simulink model "TENSGwithGFM_electromechanical"  (R2020a)
settings: Solver=VariableStepAuto  StartTime=0.0  StopTime=10.0  FixedStep=0.01  RelTol=1e-3
values from neighbouring files (symbols this model uses):
  GFMInit = GFMSimple_init(resultsac,GFM_in_gidx)    [init.m]
  GSGInit =     [SixGFMconfig.mat]    (also in eightGFMconfig.mat; fourGFMconfig.mat; init.m = SG_init(resultsac,SG_in_gidx); tenGFMconfig.mat)
  Pload = [0 0 0 0 0 0 0 0 0 0 0 0 ... (39 elements, 39x1)]    [SixGFMconfig.mat]    (also in eightGFMconfig.mat; fourGFMconfig.mat; init.m = -resultsac.bus{[CZno,CPno],3}/1000; tenGFMconfig.mat)
  Qload = -resultsac.bus{[CZno,CPno],4}/1000    [init.m]
  Satura = Ses_g(GFM_in_gidx)    [init.m]
  U = [1.0278659059 0.919047677638 0.824047236404 0.914672565668 0.984993620745 0.992890253418 1.00337242347 1.00687710353 1.06162588537 0.973548635627 0.980333735458 0.971076509646 ... (88 elements, 88x1)]    [SixGFMconfig.mat]    (also in eightGFMconfig.mat; fourGFMconfig.mat; init.m = resultsac.bus{:,8}.*exp(1i*(resultsac.bus{:,9})/180*pi); tenGFMconfig.mat)
  Vload = Vbus([CZno,CPno])    [init.m]
  W0 = wB    (= 314.159265359)    [init.m]
  Y_new = [-5.55111512313e-17 -2.77555756156e-17 0 0 0 0 0 0 0 0 0 0 ... (7744 elements, 88x88)]    [SixGFMconfig.mat]    (also in eightGFMconfig.mat; fourGFMconfig.mat; init.m = Y_new([CSno,CPno,GFMother],[CSno,CPno,GFMother]); kron.m = Y)
libraries: eeTransforms x45, simulink_extras x10
(part 1 of 3)
settings Model: Creator=Qiufan_Yang  LastModifiedBy=Qiufan_Yang
settings SolverCC: ZeroCrossAlgorithm=Adaptive
settings DebuggingCC: IgnoredZcDiagnostic=none

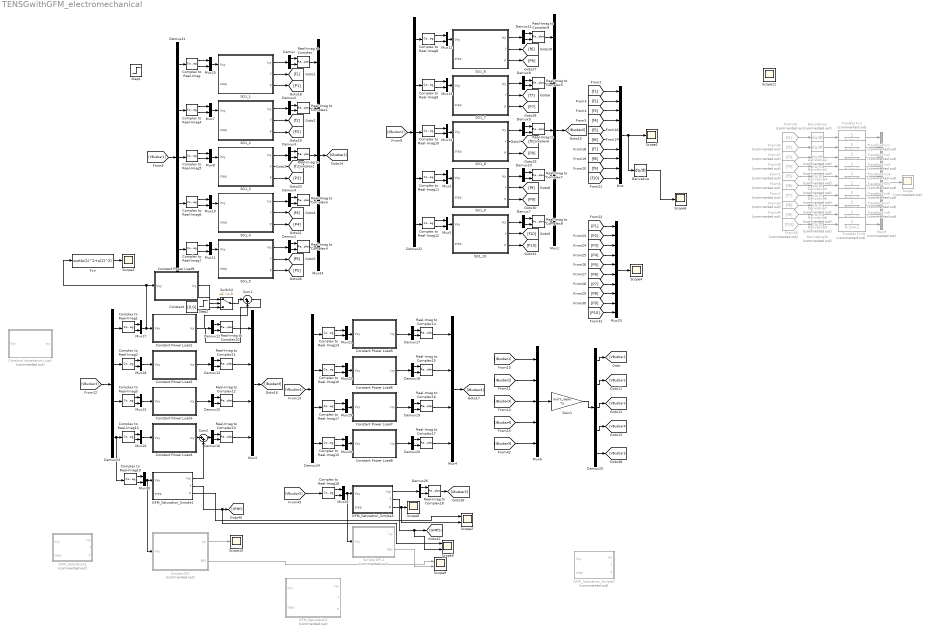
== system TENSGwithGFM_electromechanical ==
  Complex to Real-Imag{,1..19} (20 alike) : ComplexToRealImag
  Constant : Constant  Value=[0,0]
  Constant Impedance Load : Subsystem  Commented=on  mask{Pload=Pload(1), Qload=Qload(1), Vout=Vload(1), Ix0=0, Iy0=0, YLD=0}
      mask init:
      | YLD=(Pload-1j*Qload)/(abs(Vout))^2;
  Constant Power Load1 : Subsystem  mask{Pload=Pload(1), Qload=Qload(1), Vout=Vload(1), Ix0=0, Iy0=0}
      mask init:
      | Ixy=(Pload-1j*Qload)/conj(Vout);
      | Ix0=real(Ixy);
      | Iy0=imag(Ixy);
  Constant Power Load2 : Subsystem  mask{Pload=Pload(2), Qload=Qload(2), Vout=Vload(2), Ix0=0, Iy0=0}
      mask init:
      | Ixy=(Pload-1j*Qload)/conj(Vout);
      | Ix0=real(Ixy);
      | Iy0=imag(Ixy);
  Constant Power Load3 : Subsystem  mask{Pload=Pload(3), Qload=Qload(3), Vout=Vload(3), Ix0=0, Iy0=0}
      mask init:
      | Ixy=(Pload-1j*Qload)/conj(Vout);
      | Ix0=real(Ixy);
      | Iy0=imag(Ixy);
  Constant Power Load4 : Subsystem  mask{Pload=Pload(4), Qload=Qload(4), Vout=Vload(4), Ix0=0, Iy0=0}
      mask init:
      | Ixy=(Pload-1j*Qload)/conj(Vout);
      | Ix0=real(Ixy);
      | Iy0=imag(Ixy);
  Constant Power Load5 : Subsystem  mask{Pload=Pload(5), Qload=Qload(5), Vout=Vload(5), Ix0=0, Iy0=0}
      mask init:
      | Ixy=(Pload-1j*Qload)/conj(Vout);
      | Ix0=real(Ixy);
      | Iy0=imag(Ixy);
  Constant Power Load6 : Subsystem  mask{Pload=Pload(6), Qload=Qload(6), Vout=Vload(6), Ix0=0, Iy0=0}
      mask init:
      | Ixy=(Pload-1j*Qload)/conj(Vout);
      | Ix0=real(Ixy);
      | Iy0=imag(Ixy);
  Constant Power Load7 : Subsystem  mask{Pload=Pload(7), Qload=Qload(7), Vout=Vload(7), Ix0=0, Iy0=0}
      mask init:
      | Ixy=(Pload-1j*Qload)/conj(Vout);
      | Ix0=real(Ixy);
      | Iy0=imag(Ixy);
  Constant Power Load8 : Subsystem  mask{Pload=Pload(8), Qload=Qload(8), Vout=Vload(8), Ix0=0, Iy0=0}
      mask init:
      | Ixy=(Pload-1j*Qload)/conj(Vout);
      | Ix0=real(Ixy);
      | Iy0=imag(Ixy);
  Constant Power Load9 : Subsystem  mask{Pload=-0.2, Qload=0, Vout=Vload(1), Ix0=0, Iy0=0}
      mask init:
      | Ixy=(Pload-1j*Qload)/conj(Vout);
      | Ix0=real(Ixy);
      | Iy0=imag(Ixy);
  Demux{,1..4,7..13,15..20,26} (19 alike) : Demux  Outputs=2
  Demux21 : Demux  Outputs=5
  Demux22 : Demux  Outputs=5
  Demux23 : Demux
  Demux24 : Demux
  Demux25 : Demux  Outputs=[5 5 4 4 1]
  Derivative : Derivative  CoefficientInTFapproximation=1
  Derivative{1..10} (10 alike) : Derivative  Commented=on
  Fcn : Fcn  Expr=sqrt(u(1)^2+u(2)^2)
  From1 : From  Commented=on  GotoTag=f5
  From32 : From  Commented=on  GotoTag=f8
  From33 : From  Commented=on  GotoTag=f1
  From34 : From  Commented=on  GotoTag=f9
  From35 : From  Commented=on  GotoTag=f10
  From36 : From  Commented=on  GotoTag=f2
  From37 : From  Commented=on  GotoTag=f3
  From38 : From  Commented=on  GotoTag=f4
  From6 : From  Commented=on  GotoTag=f6
  From7 : From  Commented=on  GotoTag=f7
  GFM_Saturation1 : Subsystem  Commented=on  mask{Pout=1, Qout=0, Vout=1, RG=GFMInit.RG(1), LG=GFMInit.LG(1), CF=GFMInit.CF(1), LF=GFMInit.LF(1), RF=GFMInit.RF(1), JGFM=GFMInit.J(1), DGFM=GFMInit.D(1), KPV=GFMInit.KPV(1), KIV=GFMInit.KIV(1), KIF=GFMInit.KIF(1), KPC=GFMInit.KPC(1), KIC=GFMInit.KIC(1), KVF=GFMInit.KVF(1), TVF=GFMInit.TVF(1), Pref=GFMInit.Pref(1), Qref=GFMInit.Qref(1), Vd0=GFMInit.Vd0(1), theta0=GFMInit.theta0(1), Ix0=GFMInit.Ix0(1), Iy0=GFMInit.Iy0(1), Vx0=GFMInit.Vx0(1), Vy0=GFMInit.Vy0(1), IOx0=GFMInit.IOx0(1), IOy0=GFMInit.IOy0(1), Idref0=GFMInit.Idref0(1), Iqref0=GFMInit.Iqref0(1), Ed0=GFMInit.Ed0(1), Eq0=GFMInit.Eq0(1), Plimit=Satura(1)*1000, Qreflimit=0, KPLlimit=0.16*10, KILlimit=13.26, Ix0_copy=0.5, Iy0_copy=10}
      mask prompts: Qreflimit "Qlimit"; Ix0_copy "KPPlimit"; Iy0_copy "KIPlimit"
      mask init:
      | %IOxy0 = (Pout - 1i*Qout)/conj(Vout);
      | %Vxy0  = Vout + IOxy0*(RG+1i*LG);
      | %Ixy0  = IOxy0 + Vxy0*(1i*CF);
      | %Exy0  = Vxy0 + Ixy0*(RF+1i*LF);
      | 
      | %IOx0 = real(IOxy0);
      | % IOy0 = imag(IOxy0);
      | % Vx0 = real(Vxy0);
      | % Vy0 = imag(Vxy0);
      | % Ix0 = real(Ixy0);
      | % Iy0 = imag(Ixy0);
      | % Pref = real(Vxy0*conj(IOxy0));
      | % Qref = imag(Vxy0*conj(IOxy0));
      | % Vd0  = abs(Vxy0);
      | % theta0 = angle(Vxy0);
      | % 
      | % Edq0 = abs(Exy0)*exp(1i*(angle(Exy0)-theta0));
      | % Idq0 = abs(Ixy0)*exp(1i*(angle(Ixy0)-theta0));
      | % IOdq0 = abs(IOxy0)*exp(1i*(angle(IOxy0)-theta0));
      | % 
      | % temp = Edq0 - KVF*Vd0 - Idq0*(1i*LF);
      | % Ed0 = real(temp);
      | % Eq0 = imag(temp);
      | % 
      | % temp = Idq0 - KIF*IOdq0 - Vd0*(1i*CF);
      | % Idref0 = real(temp);
      | % Iqref0 = imag(temp);
      mask DialogControl Container8 Prompt: Parameters
      mask DialogControl Container9 Prompt: Power Flow
      mask DialogControl Container10 Prompt: LCL Parameters
      mask DialogControl Container20 Prompt: Control Parameters
      mask DialogControl Container21 Prompt: Initial Parameters
      mask DialogControl Container22 Prompt: Saturation Parameters
  GFM_Saturation2 : Subsystem  Commented=on  mask{Pout=1, Qout=0, Vout=1, RG=GFMInit.RG(2), LG=GFMInit.LG(2), CF=GFMInit.CF(2), LF=GFMInit.LF(2), RF=GFMInit.RF(2), JGFM=GFMInit.J(2), DGFM=GFMInit.D(2), KPV=GFMInit.KPV(2), KIV=GFMInit.KIV(2), KIF=GFMInit.KIF(2), KPC=GFMInit.KPC(2), KIC=GFMInit.KIC(2), KVF=GFMInit.KVF(2), TVF=GFMInit.TVF(2), Pref=GFMInit.Pref(2), Qref=GFMInit.Qref(2), Vd0=GFMInit.Vd0(2), theta0=GFMInit.theta0(2), Ix0=GFMInit.Ix0(2), Iy0=GFMInit.Iy0(2), Vx0=GFMInit.Vx0(2), Vy0=GFMInit.Vy0(2), IOx0=GFMInit.IOx0(2), IOy0=GFMInit.IOy0(2), Idref0=GFMInit.Idref0(2), Iqref0=GFMInit.Iqref0(2), Ed0=GFMInit.Ed0(2), Eq0=GFMInit.Eq0(2), Plimit=Satura(2)*1000, Qreflimit=0, KPLlimit=0.16*10, KILlimit=13.26, Ix0_copy=0.5, Iy0_copy=10}
      mask prompts: Qreflimit "Qlimit"; Ix0_copy "KPPlimit"; Iy0_copy "KIPlimit"
      mask init: same as TENSGwithGFM_electromechanical/GFM_Saturation1
      mask DialogControl Container8 Prompt: Parameters
      mask DialogControl Container9 Prompt: Power Flow
      mask DialogControl Container10 Prompt: LCL Parameters
      mask DialogControl Container20 Prompt: Control Parameters
      mask DialogControl Container21 Prompt: Initial Parameters
      mask DialogControl Container22 Prompt: Saturation Parameters
  GFM_Saturation_Simple1 : Subsystem  mask{Pout=0, Qout=0, Vout=Vload(4), Pref=0, theta0=GFMInit.theta0(1), EQ=GFMInit.EQ(1), LG=GFMInit.LG(1), JGFM=GFMInit.J(1)*0+0.5742, DGFM=GFMInit.D(1), Plimit=Satura(1)*0+0.05742, Qreflimit=0, KPLlimit=0.16*10, KILlimit=13.26, Ix0_copy=0.5, Iy0_copy=10}
      mask prompts: Qreflimit "Qlimit"; Ix0_copy "KPPlimit"; Iy0_copy "KIPlimit"
      mask init: same as TENSGwithGFM_electromechanical/GFM_Saturation1
      mask DialogControl Container8 Prompt: Parameters
      mask DialogControl Container9 Prompt: Power Flow
      mask DialogControl Container10 Prompt: LCL Parameters
      mask DialogControl Container20 Prompt: Control Parameters
      mask DialogControl Container22 Prompt: Saturation Parameters
  GFM_Saturation_Simple2 : Subsystem  Commented=on  mask{Pout=1, Qout=0, Vout=1, RG=GFMInit.RG(2), LG=GFMInit.LG(2), CF=GFMInit.CF(2), LF=GFMInit.LF(2), RF=GFMInit.RF(2), JGFM=GFMInit.J(2), DGFM=GFMInit.D(2), KPV=GFMInit.KPV(2), KIV=GFMInit.KIV(2), KIF=GFMInit.KIF(2), KPC=GFMInit.KPC(2), KIC=GFMInit.KIC(2), KVF=GFMInit.KVF(2), TVF=GFMInit.TVF(2), Pref=GFMInit.Pref(2), Qref=GFMInit.Qref(2), Vd0=GFMInit.Vd0(2), theta0=GFMInit.theta0(2), Ix0=GFMInit.Ix0(2), Iy0=GFMInit.Iy0(2), Vx0=GFMInit.Vx0(2), Vy0=GFMInit.Vy0(2), IOx0=GFMInit.IOx0(2), IOy0=GFMInit.IOy0(2), Idref0=GFMInit.Idref0(2), Iqref0=GFMInit.Iqref0(2), Ed0=GFMInit.Ed0(2), Eq0=GFMInit.Eq0(2), Plimit=Satura(2)*1000, Qreflimit=0, KPLlimit=0.16*10, KILlimit=13.26, Ix0_copy=0.5, Iy0_copy=10}
      mask prompts: Qreflimit "Qlimit"; Ix0_copy "KPPlimit"; Iy0_copy "KIPlimit"
      mask init: same as TENSGwithGFM_electromechanical/GFM_Saturation1
      mask DialogControl Container8 Prompt: Parameters
      mask DialogControl Container9 Prompt: Power Flow
      mask DialogControl Container10 Prompt: LCL Parameters
      mask DialogControl Container20 Prompt: Control Parameters
      mask DialogControl Container21 Prompt: Initial Parameters
      mask DialogControl Container22 Prompt: Saturation Parameters
  GFM_Saturation_Simple3 : Subsystem  mask{Pout=0, Qout=0, Vout=U(22), Pref=0, theta0=GFMInit.theta0(2), EQ=GFMInit.EQ(2), LG=GFMInit.LG(2), JGFM=GFMInit.J(2)*0+0.6571, DGFM=GFMInit.D(2), Plimit=Satura(2)*0+0.059, Qreflimit=0, KPLlimit=0.16*10, KILlimit=13.26, Ix0_copy=0.5, Iy0_copy=10}
      mask prompts: Qreflimit "Qlimit"; Ix0_copy "KPPlimit"; Iy0_copy "KIPlimit"
      mask init: same as TENSGwithGFM_electromechanical/GFM_Saturation1
      mask DialogControl Container8 Prompt: Parameters
      mask DialogControl Container9 Prompt: Power Flow
      mask DialogControl Container10 Prompt: LCL Parameters
      mask DialogControl Container20 Prompt: Control Parameters
      mask DialogControl Container22 Prompt: Saturation Parameters
  Gain1 : Gain  Gain=inv(Y_new)  Multiplication=Matrix(K*u)
  Mux : Mux  Inputs=10
  Mux1 : Mux  Inputs=5
  Mux{2,5,7..8,10..22,25,29..30} (20 alike) : Mux  Inputs=2
  Mux23 : Mux  Inputs=10
  Mux24 : Mux  Inputs=5
  Mux3 : Mux
  Mux4 : Mux
  Mux6 : Mux  Inputs=5
  Mux9 : Mux  Commented=on  Inputs=10
  Real-Imag to Complex{,1..18} (19 alike) : RealImagToComplex
  SG1_1 : Subsystem  mask{Pout=1, Qout=0, Vout=1, RG=0, LG=0, Xd=GSGInit.Xd(1), Xd1=GSGInit.Xd1(1), Xq=GSGInit.Xq(1), Td1=GSGInit.Td1(1), KAVR=GSGInit.KAVR(1), TAVR=GSGInit.TAVR(1), JSG=GSGInit.J(1), DSG=GSGInit.D(1), Ksg=GSGInit.Ksg(1), K1=GSGInit.K1(1), K3=GSGInit.K3(1), K5=GSGInit.K5(1), K7=GSGInit.K7(1), T1=GSGInit.T1(1), T2=GSGInit.T2(1), T3=GSGInit.T3(1), T4=GSGInit.T4(1), T5=GSGInit.T5(1), T6=GSGInit.T6(1), T7=GSGInit.T7(1), Pref=GSGInit.Pref(1), Efd0=GSGInit.Efd0(1), theta0=GSGInit.theta0(1), Eq10=GSGInit.Eq10(1), Vref0=GSGInit.Vref0(1)}
      mask init:
      | % IOxy0 = (Pout - 1i*Qout)/conj(Vout);
      | % % Vxy0  = Vout + IOxy0*(RG+1i*LG);
      | % EQ = Vout + 1i*Xq*IOxy0;
      | % 
      | % Vd = abs(Vout)*sin(angle(EQ)-angle(Vout));
      | % Vq = abs(Vout)*cos(angle(EQ)-angle(Vout));
      | % Iq = Vd/Xq;
      | % Id = abs(IOxy0)*sin(angle(EQ) - angle(IOxy0));
      | % 
      | % theta0 = angle(EQ) - pi/2; 
      | % 
      | % 
      | % Pref = real(Vout*conj(IOxy0));
      | % Qref = imag(Vout*conj(IOxy0));
      | % IOx0 = real(IOxy0);
      | % IOy0 = imag(IOxy0);
      | % 
      | % Eq10 = Vq + Id*Xd1;
      | % 
      | % Efd0 = Eq10 + Id*(Xd-Xd1);
      | % Vref0  = Efd0/KAVR+abs(Vout);
      | %Efd0 = Efd/KAVR;
      mask DialogControl Container8 Prompt: Parameters
      mask DialogControl Container9 Prompt: Power Flow
      mask DialogControl Container10 Prompt: L Parameters
      mask DialogControl Container12 Prompt: Transient Parameter
      mask DialogControl Container20 Prompt: Control Parameters
      mask DialogControl Container14 Prompt: AVR
      mask DialogControl Container16 Prompt: Swing
      mask DialogControl Container15 Prompt: Governor
      mask DialogControl Container21 Prompt: Initial Parameters
  SG1_10 : Subsystem  mask{Pout=1, Qout=0, Vout=1, RG=0, LG=0, Xd=GSGInit.Xd(10), Xd1=GSGInit.Xd1(10), Xq=GSGInit.Xq(10), Td1=GSGInit.Td1(10), KAVR=GSGInit.KAVR(10), TAVR=GSGInit.TAVR(10), JSG=GSGInit.J(10), DSG=GSGInit.D(10), Ksg=GSGInit.Ksg(10), K1=GSGInit.K1(10), K3=GSGInit.K3(10), K5=GSGInit.K5(10), K7=GSGInit.K7(10), T1=GSGInit.T1(10), T2=GSGInit.T2(10), T3=GSGInit.T3(10), T4=GSGInit.T4(10), T5=GSGInit.T5(10), T6=GSGInit.T6(10), T7=GSGInit.T7(10), Pref=GSGInit.Pref(10), Efd0=GSGInit.Efd0(10), theta0=GSGInit.theta0(10), Eq10=GSGInit.Eq10(10), Vref0=GSGInit.Vref0(10)}
      mask init: same as TENSGwithGFM_electromechanical/SG1_1
      mask DialogControl Container8 Prompt: Parameters
      mask DialogControl Container9 Prompt: Power Flow
      mask DialogControl Container10 Prompt: L Parameters
      mask DialogControl Container12 Prompt: Transient Parameter
      mask DialogControl Container20 Prompt: Control Parameters
      mask DialogControl Container14 Prompt: AVR
      mask DialogControl Container16 Prompt: Swing
      mask DialogControl Container15 Prompt: Governor
      mask DialogControl Container21 Prompt: Initial Parameters
  SG1_2 : Subsystem  mask{Pout=1, Qout=0, Vout=1, RG=0, LG=0, Xd=GSGInit.Xd(2), Xd1=GSGInit.Xd1(2), Xq=GSGInit.Xq(2), Td1=GSGInit.Td1(2), KAVR=GSGInit.KAVR(2), TAVR=GSGInit.TAVR(2), JSG=GSGInit.J(2), DSG=GSGInit.D(2), Ksg=GSGInit.Ksg(2), K1=GSGInit.K1(2), K3=GSGInit.K3(2), K5=GSGInit.K5(2), K7=GSGInit.K7(2), T1=GSGInit.T1(2), T2=GSGInit.T2(2), T3=GSGInit.T3(2), T4=GSGInit.T4(2), T5=GSGInit.T5(2), T6=GSGInit.T6(2), T7=GSGInit.T7(2), Pref=GSGInit.Pref(2), Efd0=GSGInit.Efd0(2), theta0=GSGInit.theta0(2), Eq10=GSGInit.Eq10(2), Vref0=GSGInit.Vref0(2)}
      mask init: same as TENSGwithGFM_electromechanical/SG1_1
      mask DialogControl Container8 Prompt: Parameters
      mask DialogControl Container9 Prompt: Power Flow
      mask DialogControl Container10 Prompt: L Parameters
      mask DialogControl Container12 Prompt: Transient Parameter
      mask DialogControl Container20 Prompt: Control Parameters
      mask DialogControl Container14 Prompt: AVR
      mask DialogControl Container16 Prompt: Swing
      mask DialogControl Container15 Prompt: Governor
      mask DialogControl Container21 Prompt: Initial Parameters
  SG1_3 : Subsystem  mask{Pout=1, Qout=0, Vout=1, RG=0, LG=0, Xd=GSGInit.Xd(3), Xd1=GSGInit.Xd1(3), Xq=GSGInit.Xq(3), Td1=GSGInit.Td1(3), KAVR=GSGInit.KAVR(3), TAVR=GSGInit.TAVR(3), JSG=GSGInit.J(3), DSG=GSGInit.D(3), Ksg=GSGInit.Ksg(3), K1=GSGInit.K1(3), K3=GSGInit.K3(3), K5=GSGInit.K5(3), K7=GSGInit.K7(3), T1=GSGInit.T1(3), T2=GSGInit.T2(3), T3=GSGInit.T3(3), T4=GSGInit.T4(3), T5=GSGInit.T5(3), T6=GSGInit.T6(3), T7=GSGInit.T7(3), Pref=GSGInit.Pref(3), Efd0=GSGInit.Efd0(3), theta0=GSGInit.theta0(3), Eq10=GSGInit.Eq10(3), Vref0=GSGInit.Vref0(3)}
      mask init: same as TENSGwithGFM_electromechanical/SG1_1
      mask DialogControl Container8 Prompt: Parameters
      mask DialogControl Container9 Prompt: Power Flow
      mask DialogControl Container10 Prompt: L Parameters
      mask DialogControl Container12 Prompt: Transient Parameter
      mask DialogControl Container20 Prompt: Control Parameters
      mask DialogControl Container14 Prompt: AVR
      mask DialogControl Container16 Prompt: Swing
      mask DialogControl Container15 Prompt: Governor
      mask DialogControl Container21 Prompt: Initial Parameters
  SG1_4 : Subsystem  mask{Pout=1, Qout=0, Vout=1, RG=0, LG=0, Xd=GSGInit.Xd(4), Xd1=GSGInit.Xd1(4), Xq=GSGInit.Xq(4), Td1=GSGInit.Td1(4), KAVR=GSGInit.KAVR(4), TAVR=GSGInit.TAVR(4), JSG=GSGInit.J(4), DSG=GSGInit.D(4), Ksg=GSGInit.Ksg(4), K1=GSGInit.K1(4), K3=GSGInit.K3(4), K5=GSGInit.K5(4), K7=GSGInit.K7(4), T1=GSGInit.T1(4), T2=GSGInit.T2(4), T3=GSGInit.T3(4), T4=GSGInit.T4(4), T5=GSGInit.T5(4), T6=GSGInit.T6(4), T7=GSGInit.T7(4), Pref=GSGInit.Pref(4), Efd0=GSGInit.Efd0(4), theta0=GSGInit.theta0(4), Eq10=GSGInit.Eq10(4), Vref0=GSGInit.Vref0(4)}
      mask init: same as TENSGwithGFM_electromechanical/SG1_1
      mask DialogControl Container8 Prompt: Parameters
      mask DialogControl Container9 Prompt: Power Flow
      mask DialogControl Container10 Prompt: L Parameters
      mask DialogControl Container12 Prompt: Transient Parameter
      mask DialogControl Container20 Prompt: Control Parameters
      mask DialogControl Container14 Prompt: AVR
      mask DialogControl Container16 Prompt: Swing
      mask DialogControl Container15 Prompt: Governor
      mask DialogControl Container21 Prompt: Initial Parameters
  SG1_5 : Subsystem  mask{Pout=1, Qout=0, Vout=1, RG=0, LG=0, Xd=GSGInit.Xd(5), Xd1=GSGInit.Xd1(5), Xq=GSGInit.Xq(5), Td1=GSGInit.Td1(5), KAVR=GSGInit.KAVR(5), TAVR=GSGInit.TAVR(5), JSG=GSGInit.J(5), DSG=GSGInit.D(5), Ksg=GSGInit.Ksg(5), K1=GSGInit.K1(5), K3=GSGInit.K3(5), K5=GSGInit.K5(5), K7=GSGInit.K7(5), T1=GSGInit.T1(5), T2=GSGInit.T2(5), T3=GSGInit.T3(5), T4=GSGInit.T4(5), T5=GSGInit.T5(5), T6=GSGInit.T6(5), T7=GSGInit.T7(5), Pref=GSGInit.Pref(5), Efd0=GSGInit.Efd0(5), theta0=GSGInit.theta0(5), Eq10=GSGInit.Eq10(5), Vref0=GSGInit.Vref0(5)}
      mask init: same as TENSGwithGFM_electromechanical/SG1_1
      mask DialogControl Container8 Prompt: Parameters
      mask DialogControl Container9 Prompt: Power Flow
      mask DialogControl Container10 Prompt: L Parameters
      mask DialogControl Container12 Prompt: Transient Parameter
      mask DialogControl Container20 Prompt: Control Parameters
      mask DialogControl Container14 Prompt: AVR
      mask DialogControl Container16 Prompt: Swing
      mask DialogControl Container15 Prompt: Governor
      mask DialogControl Container21 Prompt: Initial Parameters
  SG1_6 : Subsystem  mask{Pout=1, Qout=0, Vout=1, RG=0, LG=0, Xd=GSGInit.Xd(6), Xd1=GSGInit.Xd1(6), Xq=GSGInit.Xq(6), Td1=GSGInit.Td1(6), KAVR=GSGInit.KAVR(6), TAVR=GSGInit.TAVR(6), JSG=GSGInit.J(6), DSG=GSGInit.D(6), Ksg=GSGInit.Ksg(6), K1=GSGInit.K1(6), K3=GSGInit.K3(6), K5=GSGInit.K5(6), K7=GSGInit.K7(6), T1=GSGInit.T1(6), T2=GSGInit.T2(6), T3=GSGInit.T3(6), T4=GSGInit.T4(6), T5=GSGInit.T5(6), T6=GSGInit.T6(6), T7=GSGInit.T7(6), Pref=GSGInit.Pref(6), Efd0=GSGInit.Efd0(6), theta0=GSGInit.theta0(6), Eq10=GSGInit.Eq10(6), Vref0=GSGInit.Vref0(6)}
      mask init: same as TENSGwithGFM_electromechanical/SG1_1
      mask DialogControl Container8 Prompt: Parameters
      mask DialogControl Container9 Prompt: Power Flow
      mask DialogControl Container10 Prompt: L Parameters
      mask DialogControl Container12 Prompt: Transient Parameter
      mask DialogControl Container20 Prompt: Control Parameters
      mask DialogControl Container14 Prompt: AVR
      mask DialogControl Container16 Prompt: Swing
      mask DialogControl Container15 Prompt: Governor
      mask DialogControl Container21 Prompt: Initial Parameters
  SG1_7 : Subsystem  mask{Pout=1, Qout=0, Vout=1, RG=0, LG=0, Xd=GSGInit.Xd(7), Xd1=GSGInit.Xd1(7), Xq=GSGInit.Xq(7), Td1=GSGInit.Td1(7), KAVR=GSGInit.KAVR(7), TAVR=GSGInit.TAVR(7), JSG=GSGInit.J(7), DSG=GSGInit.D(7), Ksg=GSGInit.Ksg(7), K1=GSGInit.K1(7), K3=GSGInit.K3(7), K5=GSGInit.K5(7), K7=GSGInit.K7(7), T1=GSGInit.T1(7), T2=GSGInit.T2(7), T3=GSGInit.T3(7), T4=GSGInit.T4(7), T5=GSGInit.T5(7), T6=GSGInit.T6(7), T7=GSGInit.T7(7), Pref=GSGInit.Pref(7), Efd0=GSGInit.Efd0(7), theta0=GSGInit.theta0(7), Eq10=GSGInit.Eq10(7), Vref0=GSGInit.Vref0(7)}
      mask init: same as TENSGwithGFM_electromechanical/SG1_1
      mask DialogControl Container8 Prompt: Parameters
      mask DialogControl Container9 Prompt: Power Flow
      mask DialogControl Container10 Prompt: L Parameters
      mask DialogControl Container12 Prompt: Transient Parameter
      mask DialogControl Container20 Prompt: Control Parameters
      mask DialogControl Container14 Prompt: AVR
      mask DialogControl Container16 Prompt: Swing
      mask DialogControl Container15 Prompt: Governor
      mask DialogControl Container21 Prompt: Initial Parameters
  SG1_8 : Subsystem  mask{Pout=1, Qout=0, Vout=1, RG=0, LG=0, Xd=GSGInit.Xd(8), Xd1=GSGInit.Xd1(8), Xq=GSGInit.Xq(8), Td1=GSGInit.Td1(8), KAVR=GSGInit.KAVR(8), TAVR=GSGInit.TAVR(8), JSG=GSGInit.J(8), DSG=GSGInit.D(8), Ksg=GSGInit.Ksg(8), K1=GSGInit.K1(8), K3=GSGInit.K3(8), K5=GSGInit.K5(8), K7=GSGInit.K7(8), T1=GSGInit.T1(8), T2=GSGInit.T2(8), T3=GSGInit.T3(8), T4=GSGInit.T4(8), T5=GSGInit.T5(8), T6=GSGInit.T6(8), T7=GSGInit.T7(8), Pref=GSGInit.Pref(8), Efd0=GSGInit.Efd0(8), theta0=GSGInit.theta0(8), Eq10=GSGInit.Eq10(8), Vref0=GSGInit.Vref0(8)}
      mask init: same as TENSGwithGFM_electromechanical/SG1_1
      mask DialogControl Container8 Prompt: Parameters
      mask DialogControl Container9 Prompt: Power Flow
      mask DialogControl Container10 Prompt: L Parameters
      mask DialogControl Container12 Prompt: Transient Parameter
      mask DialogControl Container20 Prompt: Control Parameters
      mask DialogControl Container14 Prompt: AVR
      mask DialogControl Container16 Prompt: Swing
      mask DialogControl Container15 Prompt: Governor
      mask DialogControl Container21 Prompt: Initial Parameters
  SG1_9 : Subsystem  mask{Pout=1, Qout=0, Vout=1, RG=0, LG=0, Xd=GSGInit.Xd(9), Xd1=GSGInit.Xd1(9), Xq=GSGInit.Xq(9), Td1=GSGInit.Td1(9), KAVR=GSGInit.KAVR(9), TAVR=GSGInit.TAVR(9), JSG=GSGInit.J(9), DSG=GSGInit.D(9), Ksg=GSGInit.Ksg(9), K1=GSGInit.K1(9), K3=GSGInit.K3(9), K5=GSGInit.K5(9), K7=GSGInit.K7(9), T1=GSGInit.T1(9), T2=GSGInit.T2(9), T3=GSGInit.T3(9), T4=GSGInit.T4(9), T5=GSGInit.T5(9), T6=GSGInit.T6(9), T7=GSGInit.T7(9), Pref=GSGInit.Pref(9), Efd0=GSGInit.Efd0(9), theta0=GSGInit.theta0(9), Eq10=GSGInit.Eq10(9), Vref0=GSGInit.Vref0(9)}
      mask init: same as TENSGwithGFM_electromechanical/SG1_1
      mask DialogControl Container8 Prompt: Parameters
      mask DialogControl Container9 Prompt: Power Flow
      mask DialogControl Container10 Prompt: L Parameters
      mask DialogControl Container12 Prompt: Transient Parameter
      mask DialogControl Container20 Prompt: Control Parameters
      mask DialogControl Container14 Prompt: AVR
      mask DialogControl Container16 Prompt: Swing
      mask DialogControl Container15 Prompt: Governor
      mask DialogControl Container21 Prompt: Initial Parameters
  Scope : Scope  Commented=on
  Scope{1,3..4,6,8,10} (6 alike) : Scope
  Scope{2,5,9,11} (4 alike) : Scope  NumInputPorts=2
  Simple GFL : Subsystem  Commented=on  mask{JGFL=GFMInit.J(1)*0, DGFL=GFMInit.D(1)*0, KP=0.16, KI=3.71, TF=0.01, TD=0.01, TO=0.1, Pref=0, Qref=0, Id0=0, Iq0=0, theta=angle(Vload(4))}
  Simple GFL1 : Subsystem  Commented=on  mask{JGFL=GFMInit.J(2)*0, DGFL=GFMInit.D(2)*0, KP=0.16, KI=3.71, TF=0.01, TD=0.01, TO=0.1, Pref=0, Qref=0, Id0=0, Iq0=0, theta=angle(U(22))}
  Step1 : Step  After=-0.1  SampleTime=0
  Step2 : Step  SampleTime=0
  Sum1 : Sum  Inputs=|++
  Sum2 : Sum  Inputs=|++
  Switch2 : Switch  Criteria=u2 ~= 0  Threshold=0.5  SaturateOnIntegerOverflow=on
  Transfer Fcn{,1..9} (10 alike) : TransferFcn  Commented=on  Denominator=[0.1 1]
  wires:
  SG1_1/1(Ixy) -> Demux/1
  SG1_4/1(Ixy) -> Demux4/1
  Real-Imag to Complex/1 -> Mux24/1
  Real-Imag to Complex3/1 -> Mux24/4
  SG1_1/2(f) -> [f1]
  Demux/2 -> Real-Imag to Complex/2
  SG1_3/1(Ixy) -> Demux3/1
  SG1_1/3(P) -> [P1]
  Demux4/1 -> Real-Imag to Complex3/1
  Demux2/2 -> Real-Imag to Complex1/2
  Real-Imag to Complex1/1 -> Mux24/2
  Demux/1 -> Real-Imag to Complex/1
  Real-Imag to Complex2/1 -> Mux24/3
  Demux2/1 -> Real-Imag to Complex1/1
  Demux3/2 -> Real-Imag to Complex2/2
  SG1_2/1(Ixy) -> Demux2/1
  Demux4/2 -> Real-Imag to Complex3/2
  Demux3/1 -> Real-Imag to Complex2/1
  SG1_2/2(f) -> [f2]
  SG1_3/2(f) -> [f3]
  SG1_4/2(f) -> [f4]
  [f1] -> Mux/1
  [f2] -> Mux/2
  [f3] -> Mux/3
  [f4] -> Mux/4
  Mux/1 -> Derivative/1, Scope1/1
  SG1_5/2(f) -> [f5]
  SG1_5/1(Ixy) -> Demux1/1
  Demux1/2 -> Real-Imag to Complex4/2
  Demux1/1 -> Real-Imag to Complex4/1
  Real-Imag to Complex4/1 -> Mux24/5
  SG1_10/2(f) -> [f10]
  SG1_9/1(Ixy) -> Demux10/1
  SG1_8/1(Ixy) -> Demux9/1
  SG1_8/2(f) -> [f8]
  Demux9/1 -> Real-Imag to Complex6/1
  SG1_7/2(f) -> [f7]
  Demux10/2 -> Real-Imag to Complex7/2
  SG1_7/1(Ixy) -> Demux8/1
  Demux10/1 -> Real-Imag to Complex7/1
  Demux8/1 -> Real-Imag to Complex5/1
  Demux7/2 -> Real-Imag to Complex8/2
  Real-Imag to Complex8/1 -> Mux1/5
  Real-Imag to Complex6/1 -> Mux1/3
  Real-Imag to Complex5/1 -> Mux1/2
  Demux8/2 -> Real-Imag to Complex5/2
  Demux7/1 -> Real-Imag to Complex8/1
  SG1_10/1(Ixy) -> Demux7/1
  Demux9/2 -> Real-Imag to Complex6/2
  Real-Imag to Complex7/1 -> Mux1/4
  SG1_9/2(f) -> [f9]
  Demux11/2 -> Real-Imag to Complex9/2
  Real-Imag to Complex9/1 -> Mux1/1
  Demux11/1 -> Real-Imag to Complex9/1
  SG1_6/1(Ixy) -> Demux11/1
  SG1_6/2(f) -> [f6]
  Demux12/1 -> Real-Imag to Complex10/1
  Real-Imag to Complex10/1 -> Mux3/1
  Demux12/2 -> Real-Imag to Complex10/2
  Real-Imag to Complex11/1 -> Mux3/2
  Demux13/2 -> Real-Imag to Complex11/2
  Demux13/1 -> Real-Imag to Complex11/1
  Real-Imag to Complex12/1 -> Mux3/3
  Demux15/2 -> Real-Imag to Complex12/2
  Demux15/1 -> Real-Imag to Complex12/1
  Real-Imag to Complex13/1 -> Mux3/4
  Demux16/2 -> Real-Imag to Complex13/2
  Demux16/1 -> Real-Imag to Complex13/1
  Demux17/1 -> Real-Imag to Complex14/1
  Demux18/1 -> Real-Imag to Complex15/1
  Real-Imag to Complex15/1 -> Mux4/2
  Real-Imag to Complex14/1 -> Mux4/1
  Demux17/2 -> Real-Imag to Complex14/2
  Demux18/2 -> Real-Imag to Complex15/2
  Real-Imag to Complex16/1 -> Mux4/3
  Demux20/2 -> Real-Imag to Complex17/2
  Demux19/2 -> Real-Imag to Complex16/2
  Demux20/1 -> Real-Imag to Complex17/1
  Real-Imag to Complex17/1 -> Mux4/4
  Demux19/1 -> Real-Imag to Complex16/1
  Mux6/1 -> Gain1/1
  Gain1/1 -> Demux25/1
  Demux25/1 -> [VBusbar1]
  Demux25/2 -> [VBusbar2]
  Demux25/3 -> [VBusbar3]
  Demux25/4 -> [VBusbar4]
  [VBusbar1] -> Demux21/1
  Complex to Real-Imag/2 -> Mux25/2
  Complex to Real-Imag/1 -> Mux25/1
  Mux25/1 -> SG1_1/1(Vxy)
  Mux7/1 -> SG1_2/1(Vxy)
  Complex to Real-Imag4/2 -> Mux7/2
  Complex to Real-Imag4/1 -> Mux7/1
  Mux8/1 -> SG1_3/1(Vxy)
  Complex to Real-Imag5/2 -> Mux8/2
  Complex to Real-Imag5/1 -> Mux8/1
  Mux10/1 -> SG1_4/1(Vxy)
  Complex to Real-Imag6/2 -> Mux10/2
  Complex to Real-Imag6/1 -> Mux10/1
  Mux11/1 -> SG1_5/1(Vxy)
  Complex to Real-Imag7/2 -> Mux11/2
  Complex to Real-Imag7/1 -> Mux11/1
  Complex to Real-Imag11/2 -> Mux2/2
  Complex to Real-Imag10/2 -> Mux14/2
  Complex to Real-Imag10/1 -> Mux14/1
  Mux14/1 -> SG1_8/1(Vxy)
  Mux2/1 -> SG1_9/1(Vxy)
  Complex to Real-Imag9/2 -> Mux13/2
  Complex to Real-Imag9/1 -> Mux13/1
  Mux13/1 -> SG1_7/1(Vxy)
  Complex to Real-Imag8/1 -> Mux12/1
  Complex to Real-Imag11/1 -> Mux2/1
  Complex to Real-Imag12/1 -> Mux5/1
  Complex to Real-Imag8/2 -> Mux12/2
  Complex to Real-Imag12/2 -> Mux5/2
  Mux5/1 -> SG1_10/1(Vxy)
  Mux12/1 -> SG1_6/1(Vxy)
  [VBusbar2] -> Demux22/1
  Mux24/1 -> [IBusbar1]
  [IBusbar1] -> Mux6/1
  Mux1/1 -> [IBusbar2]
  [IBusbar2] -> Mux6/2
  Complex to Real-Imag3/2 -> Mux15/2
  Complex to Real-Imag3/1 -> Mux15/1
  Complex to Real-Imag2/2 -> Mux18/2
  Complex to Real-Imag2/1 -> Mux18/1
  Demux23/2 -> Complex to Real-Imag2/1
  Mux15/1 -> Constant Power Load3/1(Vxy)
  Complex to Real-Imag13/1 -> Mux16/1
  Demux23/1 -> Complex to Real-Imag1/1
  Complex to Real-Imag13/2 -> Mux16/2
  Demux23/3 -> Complex to Real-Imag3/1
  Complex to Real-Imag1/2 -> Mux17/2
  Mux16/1 -> Constant Power Load4/1(Vxy)
  Complex to Real-Imag1/1 -> Mux17/1
  [VBusbar3] -> Demux23/1
  Demux24/2 -> Complex to Real-Imag16/1
  Mux20/1 -> Constant Power Load8/1(Vxy)
  Demux24/1 -> Complex to Real-Imag14/1
  Complex to Real-Imag14/1 -> Mux21/1
  Complex to Real-Imag14/2 -> Mux21/2
  Complex to Real-Imag15/1 -> Mux20/1
  Complex to Real-Imag16/1 -> Mux22/1
  Mux22/1 -> Constant Power Load6/1(Vxy)
  Complex to Real-Imag17/2 -> Mux19/2
  Complex to Real-Imag15/2 -> Mux20/2
  Demux24/3 -> Complex to Real-Imag17/1
  Complex to Real-Imag17/1 -> Mux19/1
  Mux19/1 -> Constant Power Load7/1(Vxy)
  Complex to Real-Imag16/2 -> Mux22/2
  [VBusbar4] -> Demux24/1
  Mux3/1 -> [IBusbar3]
  Mux4/1 -> [IBusbar4]
  [IBusbar3] -> Mux6/3
  [IBusbar4] -> Mux6/4
  [f5] -> Mux/5
  [f6] -> Mux/6
  [f7] -> Mux/7
  [f8] -> Mux/8
  [f9] -> Mux/9
  [f10] -> Mux/10
  Demux21/5 -> Complex to Real-Imag7/1
  Demux21/3 -> Complex to Real-Imag5/1
  Demux21/4 -> Complex to Real-Imag6/1
  Demux21/1 -> Complex to Real-Imag/1
  Demux22/1 -> Complex to Real-Imag8/1
  Demux22/2 -> Complex to Real-Imag9/1
  Demux22/3 -> Complex to Real-Imag10/1
  Demux22/4 -> Complex to Real-Imag11/1
  Demux22/5 -> Complex to Real-Imag12/1
  Demux21/2 -> Complex to Real-Imag4/1
  SG1_2/3(P) -> [P2]
  SG1_3/3(P) -> [P3]
  SG1_4/3(P) -> [P4]
  SG1_5/3(P) -> [P5]
  SG1_6/3(P) -> [P6]
  SG1_7/3(P) -> [P7]
  SG1_8/3(P) -> [P8]
  SG1_9/3(P) -> [P9]
  SG1_10/3(P) -> [P10]
  [P1] -> Mux23/1
  [P2] -> Mux23/2
  [P3] -> Mux23/3
  [P4] -> Mux23/4
  [P5] -> Mux23/5
  [P6] -> Mux23/6
  [P7] -> Mux23/7
  [P8] -> Mux23/8
  [P9] -> Mux23/9
  [P10] -> Mux23/10
  Mux23/1 -> Scope4/1
  Derivative/1 -> Scope6/1
  Fcn/1 -> Scope3/1
  Mux18/1 -> Constant Power Load2/1(Vxy)
  Mux17/1 -> Fcn/1, Constant Power Load9/1(Vxy), Constant Power Load1/1(Vxy)
  Step2/1 -> Switch2/2
  Constant Power Load9/1(Ixy) -> Switch2/1
  Constant/1 -> Switch2/3
  Switch2/1 -> Sum1/1
  Mux21/1 -> Constant Power Load5/1(Vxy)
  Constant Power Load4/1(Ixy) -> Sum2/1
  [IBusbar5] -> Mux6/5
  Demux25/5 -> [VBusbar5]
  Complex to Real-Imag18/2 -> Mux29/2
  Complex to Real-Imag18/1 -> Mux29/1
  Mux29/1 -> GFM_Saturation_Simple3/1(Vxy), Simple GFL1/1(Vxy)
  Demux26/1 -> Real-Imag to Complex18/1
  Demux26/2 -> Real-Imag to Complex18/2
  Real-Imag to Complex18/1 -> [IBusbar5]
  Demux24/4 -> Complex to Real-Imag15/1
  Demux23/4 -> Complex to Real-Imag19/1, Complex to Real-Imag13/1
  Complex to Real-Imag19/2 -> Mux30/2
  Complex to Real-Imag19/1 -> Mux30/1
  Mux30/1 -> GFM_Saturation_Simple1/1(Vxy), Simple GFL/1(Vxy)
  GFM_Saturation_Simple1/3(P) -> Scope2/1
  GFM_Saturation_Simple3/3(P) -> Scope2/2, Scope8/1
  [VBusbar5] -> Complex to Real-Imag18/1
  GFM_Saturation_Simple1/2(f) -> Scope5/1, [GFMf1]
  GFM_Saturation_Simple3/2(f) -> Scope5/2, [GFMf2]
  Simple GFL/2(PES) -> Scope9/1
  Simple GFL1/2(PES) -> Scope9/2
  ? -> Scope11/2
  From33/1 -> Derivative1/1
  From36/1 -> Derivative2/1
  From37/1 -> Derivative3/1
  From38/1 -> Derivative4/1
  From1/1 -> Derivative5/1
  From6/1 -> Derivative6/1
  From7/1 -> Derivative7/1
  From32/1 -> Derivative8/1
  From34/1 -> Derivative9/1
  From35/1 -> Derivative10/1
  Derivative1/1 -> Transfer Fcn/1
  Transfer Fcn/1 -> Mux9/1
  Derivative2/1 -> Transfer Fcn1/1
  Transfer Fcn1/1 -> Mux9/2
  Derivative3/1 -> Transfer Fcn2/1
  Transfer Fcn2/1 -> Mux9/3
  Derivative4/1 -> Transfer Fcn3/1
  Transfer Fcn3/1 -> Mux9/4
  Derivative5/1 -> Transfer Fcn4/1
  Transfer Fcn4/1 -> Mux9/5
  Derivative6/1 -> Transfer Fcn5/1
  Transfer Fcn5/1 -> Mux9/6
  Derivative7/1 -> Transfer Fcn6/1
  Transfer Fcn6/1 -> Mux9/7
  Derivative8/1 -> Transfer Fcn7/1
  Transfer Fcn7/1 -> Mux9/8
  Derivative9/1 -> Transfer Fcn8/1
  Transfer Fcn8/1 -> Mux9/9
  Derivative10/1 -> Transfer Fcn9/1
  Transfer Fcn9/1 -> Mux9/10
  Mux9/1 -> Scope/1
  Sum2/1 -> Demux16/1
  Constant Power Load5/1(Ixy) -> Demux17/1
  Constant Power Load6/1(Ixy) -> Demux18/1
  Constant Power Load7/1(Ixy) -> Demux19/1
  Constant Power Load2/1(Ixy) -> Demux13/1
  Constant Power Load3/1(Ixy) -> Demux15/1
  Simple GFL/1(Ixy) -> Scope10/1
  Constant Power Load8/1(Ixy) -> Demux20/1
  Constant Power Load1/1(Ixy) -> Sum1/2
  Sum1/1 -> Demux12/1
  GFM_Saturation_Simple1/1(Ixy) -> Sum2/2
  GFM_Saturation_Simple3/1(Ixy) -> Demux26/1

== system TENSGwithGFM_electromechanical/Constant Impedance Load ==
  Vxy : Inport
  Constant : Constant  Value=real(YLD)
  Constant1 : Constant  Value=imag(YLD)
  Demux : Demux  Outputs=2
  Fcn8 : Fcn  Expr=u(3)*u(1)-u(2)*u(4)
  Fcn9 : Fcn  Expr=(u(3)*u(2)+u(1)*u(4))
  Mux23 : Mux
  Mux24 : Mux  Inputs=2
  Ixy : Outport
  wires:
  Mux23/1 -> Fcn8/1, Fcn9/1
  Constant1/1 -> Mux23/2
  Fcn8/1 -> Mux24/1
  Fcn9/1 -> Mux24/2
  Constant/1 -> Mux23/1
  Vxy/1 -> Demux/1
  Demux/1 -> Mux23/3
  Demux/2 -> Mux23/4
  Mux24/1 -> Ixy/1

== system TENSGwithGFM_electromechanical/Constant Power Load1 ==
  Vxy : Inport
  Constant : Constant  Value=Pload
  Constant23 : Constant  Value=Qload
  Demux : Demux  Outputs=2
  Fcn8 : Fcn  Expr=(u(3)*u(1)+u(2)*u(4))/(u(3)^2+u(4)^2)
  Fcn9 : Fcn  Expr=(-u(3)*u(2)+u(1)*u(4))/(u(3)^2+u(4)^2)
  Gain8 : Gain  Gain=1/0.01
  Integrator4 : Integrator  InitialCondition=[Ix0 Iy0]
  Mux23 : Mux
  Mux24 : Mux  Inputs=2
  Sum2 : Sum  Inputs=|+-
  Ixy : Outport
  wires:
  Mux23/1 -> Fcn8/1, Fcn9/1
  Constant23/1 -> Mux23/2
  Integrator4/1 -> Ixy/1, Sum2/2
  Gain8/1 -> Integrator4/1
  Mux24/1 -> Sum2/1
  Sum2/1 -> Gain8/1
  Fcn8/1 -> Mux24/1
  Fcn9/1 -> Mux24/2
  Constant/1 -> Mux23/1
  Vxy/1 -> Demux/1
  Demux/1 -> Mux23/3
  Demux/2 -> Mux23/4

== system TENSGwithGFM_electromechanical/Constant Power Load2 ==
  Vxy : Inport
  Constant : Constant  Value=Pload
  Constant23 : Constant  Value=Qload
  Demux : Demux  Outputs=2
  Fcn8 : Fcn  Expr=(u(3)*u(1)+u(2)*u(4))/(u(3)^2+u(4)^2)
  Fcn9 : Fcn  Expr=(-u(3)*u(2)+u(1)*u(4))/(u(3)^2+u(4)^2)
  Gain8 : Gain  Gain=1/0.01
  Integrator4 : Integrator  InitialCondition=[Ix0 Iy0]
  Mux23 : Mux
  Mux24 : Mux  Inputs=2
  Sum2 : Sum  Inputs=|+-
  Ixy : Outport
  wires:
  Demux/2 -> Mux23/4
  Demux/1 -> Mux23/3
  Vxy/1 -> Demux/1
  Constant/1 -> Mux23/1
  Fcn9/1 -> Mux24/2
  Fcn8/1 -> Mux24/1
  Sum2/1 -> Gain8/1
  Mux24/1 -> Sum2/1
  Gain8/1 -> Integrator4/1
  Integrator4/1 -> Sum2/2, Ixy/1
  Constant23/1 -> Mux23/2
  Mux23/1 -> Fcn9/1, Fcn8/1

== system TENSGwithGFM_electromechanical/Constant Power Load3 ==
  Vxy : Inport
  Constant : Constant  Value=Pload
  Constant23 : Constant  Value=Qload
  Demux : Demux  Outputs=2
  Fcn8 : Fcn  Expr=(u(3)*u(1)+u(2)*u(4))/(u(3)^2+u(4)^2)
  Fcn9 : Fcn  Expr=(-u(3)*u(2)+u(1)*u(4))/(u(3)^2+u(4)^2)
  Gain8 : Gain  Gain=1/0.01
  Integrator4 : Integrator  InitialCondition=[Ix0 Iy0]
  Mux23 : Mux
  Mux24 : Mux  Inputs=2
  Sum2 : Sum  Inputs=|+-
  Ixy : Outport
  wires:
  Mux23/1 -> Fcn8/1, Fcn9/1
  Constant23/1 -> Mux23/2
  Integrator4/1 -> Ixy/1, Sum2/2
  Gain8/1 -> Integrator4/1
  Mux24/1 -> Sum2/1
  Sum2/1 -> Gain8/1
  Fcn8/1 -> Mux24/1
  Fcn9/1 -> Mux24/2
  Constant/1 -> Mux23/1
  Vxy/1 -> Demux/1
  Demux/1 -> Mux23/3
  Demux/2 -> Mux23/4

== system TENSGwithGFM_electromechanical/Constant Power Load4 ==
  Vxy : Inport
  Constant : Constant  Value=Pload
  Constant23 : Constant  Value=Qload
  Demux : Demux  Outputs=2
  Fcn8 : Fcn  Expr=(u(3)*u(1)+u(2)*u(4))/(u(3)^2+u(4)^2)
  Fcn9 : Fcn  Expr=(-u(3)*u(2)+u(1)*u(4))/(u(3)^2+u(4)^2)
  Gain8 : Gain  Gain=1/0.01
  Integrator4 : Integrator  InitialCondition=[Ix0 Iy0]
  Mux23 : Mux
  Mux24 : Mux  Inputs=2
  Sum2 : Sum  Inputs=|+-
  Ixy : Outport
  wires:
  Demux/2 -> Mux23/4
  Demux/1 -> Mux23/3
  Vxy/1 -> Demux/1
  Constant/1 -> Mux23/1
  Fcn9/1 -> Mux24/2
  Fcn8/1 -> Mux24/1
  Sum2/1 -> Gain8/1
  Mux24/1 -> Sum2/1
  Gain8/1 -> Integrator4/1
  Integrator4/1 -> Sum2/2, Ixy/1
  Constant23/1 -> Mux23/2
  Mux23/1 -> Fcn9/1, Fcn8/1

== system TENSGwithGFM_electromechanical/Constant Power Load5 ==
  Vxy : Inport
  Constant : Constant  Value=Pload
  Constant23 : Constant  Value=Qload
  Demux : Demux  Outputs=2
  Fcn8 : Fcn  Expr=(u(3)*u(1)+u(2)*u(4))/(u(3)^2+u(4)^2)
  Fcn9 : Fcn  Expr=(-u(3)*u(2)+u(1)*u(4))/(u(3)^2+u(4)^2)
  Gain8 : Gain  Gain=1/0.01
  Integrator4 : Integrator  InitialCondition=[Ix0 Iy0]
  Mux23 : Mux
  Mux24 : Mux  Inputs=2
  Sum2 : Sum  Inputs=|+-
  Ixy : Outport
  wires:
  Demux/2 -> Mux23/4
  Demux/1 -> Mux23/3
  Vxy/1 -> Demux/1
  Constant/1 -> Mux23/1
  Fcn9/1 -> Mux24/2
  Fcn8/1 -> Mux24/1
  Sum2/1 -> Gain8/1
  Mux24/1 -> Sum2/1
  Gain8/1 -> Integrator4/1
  Integrator4/1 -> Sum2/2, Ixy/1
  Constant23/1 -> Mux23/2
  Mux23/1 -> Fcn9/1, Fcn8/1

== system TENSGwithGFM_electromechanical/Constant Power Load6 ==
  Vxy : Inport
  Constant : Constant  Value=Pload
  Constant23 : Constant  Value=Qload
  Demux : Demux  Outputs=2
  Fcn8 : Fcn  Expr=(u(3)*u(1)+u(2)*u(4))/(u(3)^2+u(4)^2)
  Fcn9 : Fcn  Expr=(-u(3)*u(2)+u(1)*u(4))/(u(3)^2+u(4)^2)
  Gain8 : Gain  Gain=1/0.01
  Integrator4 : Integrator  InitialCondition=[Ix0 Iy0]
  Mux23 : Mux
  Mux24 : Mux  Inputs=2
  Sum2 : Sum  Inputs=|+-
  Ixy : Outport
  wires:
  Mux23/1 -> Fcn8/1, Fcn9/1
  Constant23/1 -> Mux23/2
  Integrator4/1 -> Ixy/1, Sum2/2
  Gain8/1 -> Integrator4/1
  Mux24/1 -> Sum2/1
  Sum2/1 -> Gain8/1
  Fcn8/1 -> Mux24/1
  Fcn9/1 -> Mux24/2
  Constant/1 -> Mux23/1
  Vxy/1 -> Demux/1
  Demux/1 -> Mux23/3
  Demux/2 -> Mux23/4

== system TENSGwithGFM_electromechanical/Constant Power Load7 ==
  Vxy : Inport
  Constant : Constant  Value=Pload
  Constant23 : Constant  Value=Qload
  Demux : Demux  Outputs=2
  Fcn8 : Fcn  Expr=(u(3)*u(1)+u(2)*u(4))/(u(3)^2+u(4)^2)
  Fcn9 : Fcn  Expr=(-u(3)*u(2)+u(1)*u(4))/(u(3)^2+u(4)^2)
  Gain8 : Gain  Gain=1/0.01
  Integrator4 : Integrator  InitialCondition=[Ix0 Iy0]
  Mux23 : Mux
  Mux24 : Mux  Inputs=2
  Sum2 : Sum  Inputs=|+-
  Ixy : Outport
  wires:
  Demux/2 -> Mux23/4
  Demux/1 -> Mux23/3
  Vxy/1 -> Demux/1
  Constant/1 -> Mux23/1
  Fcn9/1 -> Mux24/2
  Fcn8/1 -> Mux24/1
  Sum2/1 -> Gain8/1
  Mux24/1 -> Sum2/1
  Gain8/1 -> Integrator4/1
  Integrator4/1 -> Sum2/2, Ixy/1
  Constant23/1 -> Mux23/2
  Mux23/1 -> Fcn9/1, Fcn8/1

== system TENSGwithGFM_electromechanical/Constant Power Load8 ==
  Vxy : Inport
  Constant : Constant  Value=Pload
  Constant23 : Constant  Value=Qload
  Demux : Demux  Outputs=2
  Fcn8 : Fcn  Expr=(u(3)*u(1)+u(2)*u(4))/(u(3)^2+u(4)^2)
  Fcn9 : Fcn  Expr=(-u(3)*u(2)+u(1)*u(4))/(u(3)^2+u(4)^2)
  Gain8 : Gain  Gain=1/0.01
  Integrator4 : Integrator  InitialCondition=[Ix0 Iy0]
  Mux23 : Mux
  Mux24 : Mux  Inputs=2
  Sum2 : Sum  Inputs=|+-
  Ixy : Outport
  wires:
  Mux23/1 -> Fcn8/1, Fcn9/1
  Constant23/1 -> Mux23/2
  Integrator4/1 -> Ixy/1, Sum2/2
  Gain8/1 -> Integrator4/1
  Mux24/1 -> Sum2/1
  Sum2/1 -> Gain8/1
  Fcn8/1 -> Mux24/1
  Fcn9/1 -> Mux24/2
  Constant/1 -> Mux23/1
  Vxy/1 -> Demux/1
  Demux/1 -> Mux23/3
  Demux/2 -> Mux23/4

== system TENSGwithGFM_electromechanical/Constant Power Load9 ==
  Vxy : Inport
  Constant : Constant  Value=Pload
  Constant23 : Constant  Value=Qload
  Demux : Demux  Outputs=2
  Fcn8 : Fcn  Expr=(u(3)*u(1)+u(2)*u(4))/(u(3)^2+u(4)^2)
  Fcn9 : Fcn  Expr=(-u(3)*u(2)+u(1)*u(4))/(u(3)^2+u(4)^2)
  Gain8 : Gain  Gain=1/0.01
  Integrator4 : Integrator  InitialCondition=[Ix0 Iy0]
  Mux23 : Mux
  Mux24 : Mux  Inputs=2
  Sum2 : Sum  Inputs=|+-
  Ixy : Outport
  wires:
  Demux/2 -> Mux23/4
  Demux/1 -> Mux23/3
  Vxy/1 -> Demux/1
  Constant/1 -> Mux23/1
  Fcn9/1 -> Mux24/2
  Fcn8/1 -> Mux24/1
  Sum2/1 -> Gain8/1
  Mux24/1 -> Sum2/1
  Gain8/1 -> Integrator4/1
  Integrator4/1 -> Sum2/2, Ixy/1
  Constant23/1 -> Mux23/2
  Mux23/1 -> Fcn9/1, Fcn8/1

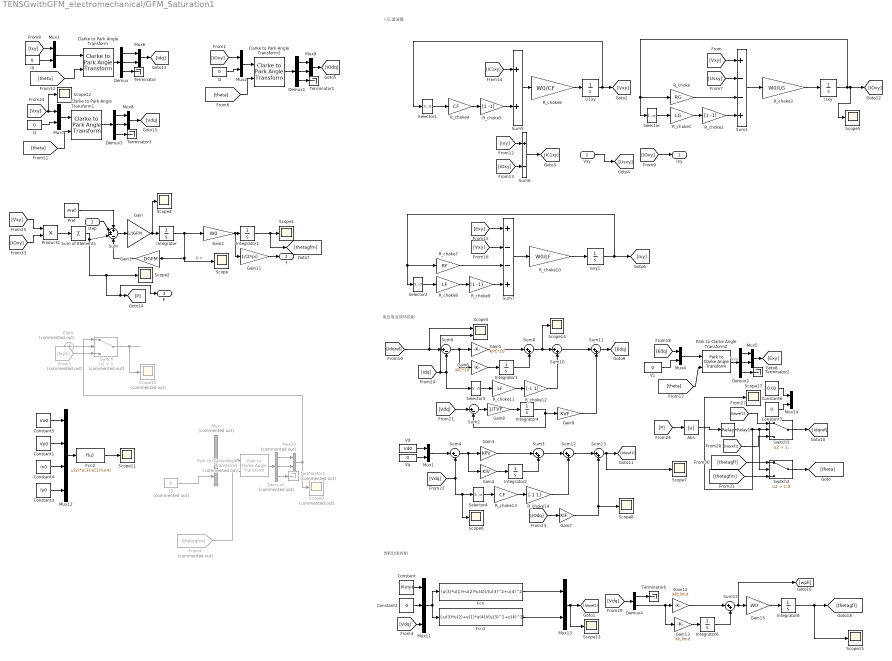
== system TENSGwithGFM_electromechanical/GFM_Saturation1 ==
  note: 饱和功率控制
  note: 电压电流双环控制
  note: LCL滤波器
  Vxy : Inport
  step : Inport  Port=2
  Abs : Abs
  Clarke to Park Angle Transform : eeTransforms/Clarke to Park Angle Transform  AxisAlignment=D-axis
      settings: SourceProductBaseCode=PS
  Clarke to Park Angle Transform1 : eeTransforms/Clarke to Park Angle Transform  AxisAlignment=D-axis
      settings: SourceProductBaseCode=PS
  Clarke to Park Angle Transform2 : eeTransforms/Clarke to Park Angle Transform  AxisAlignment=D-axis
      settings: SourceProductBaseCode=PS
  Clock : Clock  Commented=on
  Constant : Constant  Value=Plimit
  Constant1 : Constant  Value=Vy0
  Constant2 : Constant  Value=0
  Constant3 : Constant  Value=Iy0
  Constant4 : Constant  Value=Ix0
  Constant5 : Constant  Value=Vx0
  Constant6 : Constant  Value=0.02
  Constant7 : Constant  Value=0
  Demux{,1..3} (4 alike) : Demux  Outputs=3
  Demux4 : Demux  Outputs=2
  Demux5 : Demux  Commented=on  Outputs=3
  Fcn : Fcn  Expr=(u(3)*u(1)+u(2)*u(4))/(u(3)^2+u(4)^2)
  Fcn1 : Fcn  Expr=(-u(3)*u(2)+u(1)*u(4))/(u(3)^2+u(4)^2)
  Fcn2 : Fcn  Expr=u(2)*u(3)-u(1)*u(4)
  From4 : From  Commented=on  GotoTag=thetagfm
  From5 : From  Commented=on  GotoTag=Ixy1
  Gain : Gain  Gain=1/JGFM
  Gain1 : Gain  Gain=DGFM
  Gain11 : Gain  Gain=1/(2*pi)
  Gain12 : Gain  Gain=KPLlimit
  Gain13 : Gain  Gain=KILlimit
  Gain15 : Gain  Gain=W0
  Gain2 : Gain  Gain=W0
  Gain3 : Gain  Gain=KPV
  Gain4 : Gain  Gain=KIV
  Gain5 : Gain  Gain=KPC*10
  Gain6 : Gain  Gain=KIC*10
  Gain7 : Gain  Gain=KIF
  Gain8 : Gain  Gain=1/TVF
  Gain9 : Gain  Gain=KVF
  I0 : Constant  Value=0
  I1 : Constant  Value=0
  I2 : Constant  Value=0
  I3 : Constant  Commented=on  Value=0
  Integrator : Integrator
  Integrator1 : Integrator  InitialCondition=theta0
  Integrator2 : Integrator  InitialCondition=[Idref0 Iqref0]
  Integrator3 : Integrator  InitialCondition=[Ed0 Eq0]
  Integrator4 : Integrator  InitialCondition=[Vd0 0]
  Integrator6 : Integrator
  Integrator8 : Integrator  InitialCondition=theta0
  Isxy : Integrator  InitialCondition=[IOx0 IOy0]
  Isxy1 : Integrator  InitialCondition=[Ix0 Iy0]
  Mux : Mux  Commented=on  Inputs=3
  Mux{1..9,13..14} (11 alike) : Mux  Inputs=2
  Mux10 : Mux  Commented=on  Inputs=2
  Mux11 : Mux  Inputs=3
  Mux12 : Mux
  Park to Clarke Angle Transform1 : eeTransforms/Park to Clarke Angle Transform  Commented=on  AxisAlignment=D-axis
      settings: SourceProductBaseCode=PS
  Park to Clarke Angle Transform2 : eeTransforms/Park to Clarke Angle Transform  AxisAlignment=D-axis
      settings: SourceProductBaseCode=PS
  Pref : Constant  Value=Pref
  Product2 : Product
  R_choke : Gain  Gain=RG  SaturateOnIntegerOverflow=on  OutDataTypeStr=Inherit: Same as input  ParamDataTypeStr=Inherit: Same as input
  R_choke1 : Gain  Gain=LG  SaturateOnIntegerOverflow=on  OutDataTypeStr=Inherit: Same as input  ParamDataTypeStr=Inherit: Same as input
  R_choke10 : Gain  Gain=W0/LF  SaturateOnIntegerOverflow=on  OutDataTypeStr=Inherit: Same as input  ParamDataTypeStr=Inherit: Same as input
  R_choke11 : Gain  Gain=LF  SaturateOnIntegerOverflow=on  OutDataTypeStr=Inherit: Same as input  ParamDataTypeStr=Inherit: Same as input
  R_choke12 : Gain  Gain=[-1 1]  SaturateOnIntegerOverflow=on  OutDataTypeStr=Inherit: Same as input  ParamDataTypeStr=Inherit: Same as input
  R_choke13 : Gain  Gain=CF  SaturateOnIntegerOverflow=on  OutDataTypeStr=Inherit: Same as input  ParamDataTypeStr=Inherit: Same as input
  R_choke14 : Gain  Gain=[-1 1]  SaturateOnIntegerOverflow=on  OutDataTypeStr=Inherit: Same as input  ParamDataTypeStr=Inherit: Same as input
  R_choke2 : Gain  Gain=[1 -1]  SaturateOnIntegerOverflow=on  OutDataTypeStr=Inherit: Same as input  ParamDataTypeStr=Inherit: Same as input
  R_choke3 : Gain  Gain=W0/LG  SaturateOnIntegerOverflow=on  OutDataTypeStr=Inherit: Same as input  ParamDataTypeStr=Inherit: Same as input
  R_choke4 : Gain  Gain=CF  SaturateOnIntegerOverflow=on  OutDataTypeStr=Inherit: Same as input  ParamDataTypeStr=Inherit: Same as input
  R_choke5 : Gain  Gain=[1 -1]  SaturateOnIntegerOverflow=on  OutDataTypeStr=Inherit: Same as input  ParamDataTypeStr=Inherit: Same as input
  R_choke6 : Gain  Gain=W0/CF  SaturateOnIntegerOverflow=on  OutDataTypeStr=Inherit: Same as input  ParamDataTypeStr=Inherit: Same as input
  R_choke7 : Gain  Gain=RF  SaturateOnIntegerOverflow=on  OutDataTypeStr=Inherit: Same as input  ParamDataTypeStr=Inherit: Same as input
  R_choke8 : Gain  Gain=LF  SaturateOnIntegerOverflow=on  OutDataTypeStr=Inherit: Same as input  ParamDataTypeStr=Inherit: Same as input
  R_choke9 : Gain  Gain=[1 -1]  SaturateOnIntegerOverflow=on  OutDataTypeStr=Inherit: Same as input  ParamDataTypeStr=Inherit: Same as input
  Relay1 : Relay  OnSwitchValue=Plimit  OffSwitchValue=0  OnOutputValue=1.1
  Scope{,1..2,4..8,11..15,17} (14 alike) : Scope
  Scope10 : Scope  Commented=on
  Scope3 : Scope  NumInputPorts=2
  Scope9 : Scope  Commented=on
  Selector{,1..4} (5 alike) : Selector  InputPortWidth=2  IndexOptions=Index vector (dialog)  Indices=[2 1]  OutputSizes=1
  Sum : Sum  Inputs=++--
  Sum of Elements : Sum  Inputs=+
  Sum1 : Sum  Inputs=+--+  SaturateOnIntegerOverflow=on
  Sum{3,8,10..13,15} (7 alike) : Sum  Inputs=|++
  Sum2 : Sum  Inputs=|+-
  Sum4 : Sum  Inputs=|+-
  Sum5 : Sum  SaturateOnIntegerOverflow=on
  Sum6 : Sum  Inputs=+-  SaturateOnIntegerOverflow=on
  Sum7 : Sum  Inputs=+--+  SaturateOnIntegerOverflow=on
  Sum9 : Sum  Inputs=|+-
  Switch : Switch  Commented=on  Criteria=u2 > Threshold  Threshold=1
  Switch1 : Switch  Criteria=u2 > Threshold  Threshold=1.
  Switch2 : Switch  Criteria=u2 > Threshold  Threshold=1.0
  Terminator{,1..3,5} (5 alike) : Terminator
  Terminator4 : Terminator  Commented=on
  U1xy : Integrator  InitialCondition=[Vx0 Vy0]
  V1 : Constant  Value=0
  Vd : Constant  Value=Vd0
  Vq : Constant  Value=0
  Ixy : Outport
  f : Outport  Port=2
  P : Outport  Port=3
  wires:
  Integrator1/1 -> [thetagfm], Scope1/1
  Mux3/1 -> Clarke to Park Angle Transform/1
  I0/1 -> Mux3/2
  Demux/3 -> Terminator/1
  Demux/2 -> Mux6/2
  Gain/1 -> Scope4/1, Integrator/1
  Demux/1 -> Mux6/1
  Clarke to Park Angle Transform/1 -> Demux/1
  Integrator/1 -> Gain2/1, Scope/1, Gain1/1  "p.u."
  Sum of Elements/1 -> Sum/3, P/1, [P], Scope2/1
  Sum/1 -> Gain/1
  Vxy/1 -> [Usxy]
  [Vxy] -> Sum1/1
  [Usxy] -> Sum1/2
  Sum1/1 -> R_choke3/1
  R_choke3/1 -> Isxy/1
  R_choke1/1 -> R_choke2/1
  Isxy/1 -> Scope5/1, [IOxy], R_choke/1, Selector/1
  R_choke/1 -> Sum1/3
  Selector/1 -> R_choke1/1
  R_choke2/1 -> Sum1/4
  [Ixy] -> Mux3/1
  [IOxy] -> Ixy/1
  [theta] -> Clarke to Park Angle Transform/2
  Gain4/1 -> Integrator2/1
  Sum3/1 -> Sum12/1
  Gain3/1 -> Sum3/1
  Integrator2/1 -> Sum3/2
  Sum4/1 -> Gain4/1, Gain3/1
  Vd/1 -> Mux1/1
  Vq/1 -> Mux1/2
  Mux1/1 -> Sum4/1
  R_choke4/1 -> R_choke5/1
  R_choke5/1 -> Sum5/2
  Sum6/1 -> [IC1xy]
  U1xy/1 -> Selector1/1, [Vxy]
  R_choke6/1 -> U1xy/1
  [Ixy] -> Sum6/1
  Selector1/1 -> R_choke4/1
  [IOxy] -> Sum6/2
  [IC1xy] -> Sum5/1
  Sum5/1 -> R_choke6/1
  Isxy1/1 -> [Ixy], R_choke7/1, Selector2/1
  [Vxy] -> Sum7/2
  R_choke7/1 -> Sum7/3
  R_choke8/1 -> R_choke9/1
  R_choke10/1 -> Isxy1/1
  Sum7/1 -> R_choke10/1
  R_choke9/1 -> Sum7/4
  Selector2/1 -> R_choke8/1
  [Edq] -> Mux4/1
  V1/1 -> Mux4/2
  Mux4/1 -> Park to Clarke Angle Transform2/1
  [theta] -> Park to Clarke Angle Transform2/2
  Mux5/1 -> [Exy]
  Demux2/3 -> Terminator2/1
  Park to Clarke Angle Transform2/1 -> Demux2/1  "Vxy"
  Demux2/2 -> Mux5/2
  Demux2/1 -> Mux5/1
  Sum9/1 -> Gain6/1, Gain5/1
  Gain5/1 -> Sum8/1
  Gain6/1 -> Integrator3/1
  Integrator3/1 -> Sum8/2
  R_choke11/1 -> R_choke12/1
  Selector3/1 -> R_choke11/1
  Sum8/1 -> Scope14/1, Sum10/1
  R_choke12/1 -> Sum10/2
  Sum10/1 -> Sum11/1
  Gain9/1 -> Sum11/2
  Sum11/1 -> [Edq]
  Selector4/1 -> R_choke13/1
  [Vdq] -> Scope6/1, Selector4/1, Sum4/2
  R_choke13/1 -> R_choke14/1
  R_choke14/1 -> Sum12/2
  Sum12/1 -> Sum13/1
  Sum13/1 -> Scope7/1, [Idqref1]
  [IOdq] -> Gain7/1
  Gain7/1 -> Sum13/2, Scope8/1
  Mux6/1 -> [Idq]
  [Vxy] -> Scope12/1, Mux7/1
  I1/1 -> Mux7/2
  Mux7/1 -> Clarke to Park Angle Transform1/1
  [theta] -> Clarke to Park Angle Transform1/2
  Clarke to Park Angle Transform1/1 -> Demux3/1
  Demux3/1 -> Mux8/1
  Demux3/2 -> Mux8/2
  Mux8/1 -> [Vdq]
  Demux3/3 -> Terminator3/1
  [theta] -> Clarke to Park Angle Transform2/2
  Clarke to Park Angle Transform2/1 -> Demux1/1
  Demux1/1 -> Mux9/1
  Demux1/2 -> Mux9/2
  [IOxy] -> Mux2/1
  Demux1/3 -> Terminator1/1
  Mux2/1 -> Clarke to Park Angle Transform2/1
  Mux9/1 -> [IOdq]
  I2/1 -> Mux2/2
  [Vxy] -> Product2/1
  [IOxy] -> Product2/2
  Product2/1 -> Sum of Elements/1
  Sum2/1 -> Gain8/1
  Integrator4/1 -> Gain9/1, Sum2/2
  Gain8/1 -> Integrator4/1
  [Vdq] -> Sum2/1
  [Exy] -> Sum7/1
  Gain2/1 -> Gain11/1, Integrator1/1
  Gain11/1 -> f/1
  Pref/1 -> Sum/1
  [Idq] -> Sum9/2, Selector3/1, Scope3/2
  Demux5/3 -> Terminator4/1
  Mux/1 -> Park to Clarke Angle Transform1/1
  Demux5/2 -> Mux10/2
  Park to Clarke Angle Transform1/1 -> Demux5/1
  Mux10/1 -> Scope9/1, Switch/1
  Demux5/1 -> Mux10/1
  I3/1 -> Mux/3
  [Idqref] -> Scope3/1, Sum9/1
  Switch/1 -> Scope10/1
  From5/1 -> Switch/3
  Clock/1 -> Switch/2
  From4/1 -> Park to Clarke Angle Transform1/2
  Mux11/1 -> Fcn1/1, Fcn/1
  Constant/1 -> Mux11/1
  Constant5/1 -> Mux12/1
  Constant1/1 -> Mux12/2
  Constant4/1 -> Mux12/3
  Constant3/1 -> Mux12/4
  Mux12/1 -> Fcn2/1
  Constant2/1 -> Mux11/2
  Fcn2/1 -> Scope11/1
  Mux13/1 -> Scope13/1, [Idqref2]
  [P] -> Abs/1
  Relay1/1 -> Scope17/1, Switch1/2, Switch2/2
  Switch1/1 -> [Idqref]
  [Idqref1] -> Switch1/3
  Integrator6/1 -> Sum15/2
  Gain13/1 -> Integrator6/1
  Demux4/1 -> Terminator5/1
  Gain15/1 -> Integrator8/1
  [Vdq] -> Demux4/1
  Demux4/2 -> Gain13/1, Gain12/1
  Integrator8/1 -> Scope15/1, [thetagfl]
  Gain12/1 -> Sum15/1
  [thetagfl] -> Switch2/1
  [thetagfm] -> Switch2/3
  Switch2/1 -> [theta]
  Fcn/1 -> Mux13/1
  Fcn1/1 -> Mux13/2
  [Vdq] -> Mux11/3
  Constant6/1 -> Mux14/1
  Constant7/1 -> Mux14/2
  [Idqref2] -> Switch1/1
  Sum15/1 -> [wpll], Gain15/1
  Abs/1 -> Relay1/1
  Gain1/1 -> Sum/4
  step/1 -> Sum/2
